simulink model "model"  (R2022b)
settings: Solver=VariableStepAuto  StartTime=0.0  StopTime=10.0  RelTol=1e-3
values from neighbouring files (symbols this model uses):
  K1 = [kx1,0 ... (first row only)    [init_params.m]
  K2 = [kx2,0 ... (first row only)    [init_params.m]
  obj = [60,30]    [init_params.m]
  thr = 5    [init_params.m]
  X01 = [x01;y01]    [init_params.m]
  X02 = [x02;y02]    [init_params.m]
  X1d = [x1d;y1d]    [init_params.m]
  X1d_dot = [x1d_dot; y1d_dot]    [init_params.m]
  X2d = [x2d;y2d]    [init_params.m]
  X2d_dot = [x2d_dot; y2d_dot]    [init_params.m]
libraries: slctrlblks x1
settings Model: Creator=dorec  LastModifiedBy=dorec

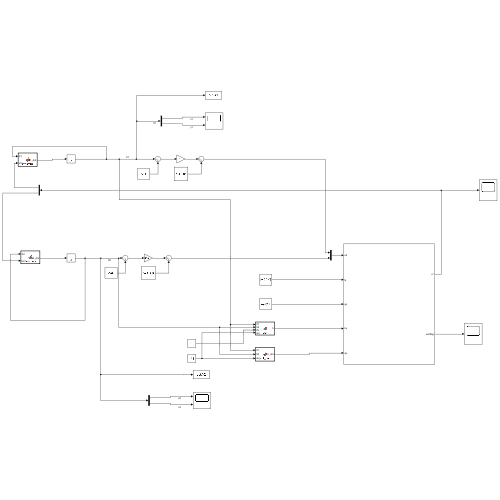
[thumbnail: Simulink's stored preview of the top-level diagram]
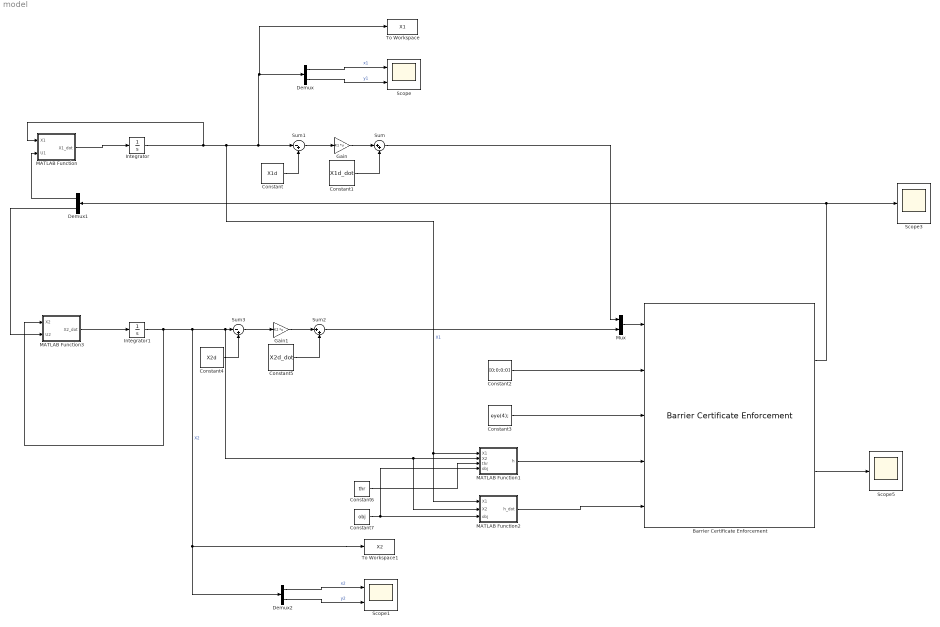
== system model ==
  Barrier Certificate Enforcement : slctrlblks/Barrier Certificate Enforcement  nx=4  nu=4  nc=3  gamma=10  beta=1  external_umax=off  external_umin=off  Ts=0.1  maxiter=200  tol=1e-6  output_exitflag=on
  Constant : Constant  Value=X1d
  Constant1 : Constant  Value=X1d_dot
  Constant2 : Constant  Value=[0;0;0;0]
  Constant3 : Constant  Value=eye(4);
  Constant4 : Constant  Value=X2d
  Constant5 : Constant  Value=X2d_dot
  Constant6 : Constant  Value=thr
  Constant7 : Constant  Value=obj
  Demux : Demux  Outputs=2
  Demux1 : Demux  Outputs=2
  Demux2 : Demux  Outputs=2
  Gain : Gain  Gain=K1  Multiplication=Matrix(K*u)
  Gain1 : Gain  Gain=K2  Multiplication=Matrix(K*u)
  Integrator : Integrator  InitialCondition=X01
  Integrator1 : Integrator  InitialCondition=X02
  MATLAB Function : MATLAB Function  TreatAsAtomicUnit=on
  MATLAB Function1 : MATLAB Function  TreatAsAtomicUnit=on
  MATLAB Function2 : MATLAB Function  TreatAsAtomicUnit=on
  MATLAB Function3 : MATLAB Function  TreatAsAtomicUnit=on
  Mux : Mux  Inputs=2
  Scope : Scope  NumInputPorts=2
  Scope1 : Scope  NumInputPorts=2
  Scope3 : Scope
  Scope5 : Scope
  Sum : Sum  Inputs=|++
  Sum1 : Sum  Inputs=|-+
  Sum2 : Sum  Inputs=|++
  Sum3 : Sum  Inputs=|-+
  To Workspace : ToWorkspace  VariableName=X1  SaveFormat=Timeseries  SampleTime=-1
  To Workspace1 : ToWorkspace  VariableName=X2  SaveFormat=Timeseries  SampleTime=-1
  wires:
  Integrator/1 -> MATLAB Function2/1(X1), MATLAB Function1/1(X1), Sum1/1, To Workspace/1, Demux/1, MATLAB Function/1(X1)  "X1"
  Sum1/1 -> Gain/1
  Constant/1 -> Sum1/2
  Gain/1 -> Sum/1
  Constant1/1 -> Sum/2
  Sum/1 -> Mux/1
  MATLAB Function/1(X1_dot) -> Integrator/1
  Demux/1 -> Scope/1  "x1"
  Demux/2 -> Scope/2  "y1"
  MATLAB Function1/1(h) -> Barrier Certificate Enforcement/4
  MATLAB Function2/1(h_dot) -> Barrier Certificate Enforcement/5
  Constant3/1 -> Barrier Certificate Enforcement/3
  Constant2/1 -> Barrier Certificate Enforcement/2
  Barrier Certificate Enforcement/1 -> Scope3/1, Demux1/1
  Constant5/1 -> Sum2/2
  Constant4/1 -> Sum3/2
  Gain1/1 -> Sum2/1
  Sum3/1 -> Gain1/1
  Integrator1/1 -> MATLAB Function3/1(X2), To Workspace1/1, Demux2/1, MATLAB Function2/2(X2), MATLAB Function1/2(X2), Sum3/1  "X2"
  MATLAB Function3/1(X2_dot) -> Integrator1/1
  Sum2/1 -> Mux/2
  Mux/1 -> Barrier Certificate Enforcement/1
  Demux1/1 -> MATLAB Function/2(U1)
  Demux1/2 -> MATLAB Function3/2(U2)
  Demux2/1 -> Scope1/1  "x2"
  Demux2/2 -> Scope1/2  "y2"
  Barrier Certificate Enforcement/2 -> Scope5/1
  Constant6/1 -> MATLAB Function1/3(thr)
  Constant7/1 -> MATLAB Function2/3(obj), MATLAB Function1/4(obj)

== matlab function model/MATLAB Function1 ==
  data: X1 input; X2 input; thr input; h output; obj input
function h = cbf(X1, X2, thr, obj)

h1 = norm(X1 - X2) - thr;
h2 = norm(X1 - obj) - thr;
h3 = norm(X2 - obj) - thr;

% if h1 <= h2
%     h = h1;
%     mem = 0;
% else
%     h = h2;
%     mem = 1;
% end
% 
% if h3 <= h
%     h = h3;
%     mem = 2;
% end

h = [h1; h2; h3];
% mem = 0;

== matlab function model/MATLAB Function ==
  data: X1 input; U1 input size=[2 1]; X1_dot output
function X1_dot = dynamics(X1,U1)

x1_dot = U1(1);
y1_dot = U1(2);

X1_dot = [x1_dot; y1_dot];

== matlab function model/MATLAB Function2 ==
  data: X1 input; X2 input; obj input; h_dot output
function h_dot = cbf_dot(X1, X2, obj)

% if mem == 1
%     h_dot = [(X1(1)-obj(1))/norm(X1-obj), (X1(2)-obj(2))/norm(X1-obj), 0, 0];
% elseif mem == 2
%     h_dot = [0, 0, (X2(1)-obj(1))/norm(X2-obj), (X2(2)-obj(2))/norm(X2-obj)];
% else
%     h_dot = [(X1(1)-X2(1))/norm(X1-X2), (X1(2)-X2(2))/norm(X1-X2), -(X1(1)-X2(1))/norm(X1-X2), -(X1(2)-X2(2))/norm(X1-X2)];
% end

h_dot = [(X1(1)-X2(1))/norm(X1-X2), (X1(2)-X2(2))/norm(X1-X2), -(X1(1)-X2(1))/norm(X1-X2), -(X1(2)-X2(2))/norm(X1-X2);
        (X1(1)-obj(1))/norm(X1-obj), (X1(2)-obj(2))/norm(X1-obj), 0, 0;
        0, 0, (X2(1)-obj(1))/norm(X2-obj), (X2(2)-obj(2))/norm(X2-obj)];

== matlab function model/MATLAB Function3 ==
  data: X2 input; U2 input size=[2 1]; X2_dot output
function X2_dot = dynamics(X2,U2)

x2_dot = U2(1);
y2_dot = U2(2);

X2_dot = [x2_dot; y2_dot];
